simulink model "train_sim"  (R2020b)
settings: Solver=VariableStepAuto  StartTime=0.0  StopTime=10.0  RelTol=1e-3
settings Model: Creator=lima  LastModifiedBy=lima

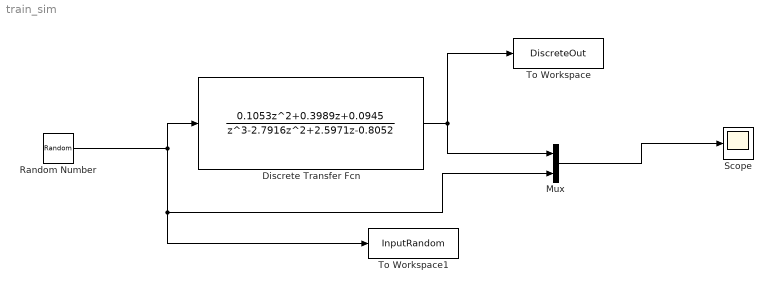
== system train_sim ==
  Discrete Transfer Fcn : DiscreteTransferFcn  Numerator="[0    0.1053    0.3989    0.0945]"  Denominator="[1.0000   -2.7916    2.5971   -0.8052]"
  Mux : Mux  Inputs=2
  Random Number : RandomNumber  SampleTime=0.1
  Scope : Scope
  To Workspace : ToWorkspace  VariableName=DiscreteOut  SaveFormat=Timeseries  SampleTime=-1
  To Workspace1 : ToWorkspace  VariableName=InputRandom  SaveFormat=Timeseries  SampleTime=-1
  wires:
  Random Number/1 -> To Workspace1/1, Mux/2, Discrete Transfer Fcn/1
  Discrete Transfer Fcn/1 -> Mux/1, To Workspace/1
  Mux/1 -> Scope/1
